simulink model "wall_plumbing_V2"  (R2017b)
settings: Solver=VariableStepAuto  StartTime=0.0  StopTime=tf  RelTol=1e-3  AbsTol=1e-3  EnableMultiTasking=on
values from neighbouring files (symbols this model uses):
  cistern_diam = 100    [plumbing_variables.m]
  cistern_inlet_diam = 2    [plumbing_variables.m]
  cistern_outlet_diam = 2    [plumbing_variables.m]
  random_seed = rand()    [plumbing_variables.m]
  swh_inlet_diam = 2    [plumbing_variables.m]
  swh_outlet_diam = 2    [plumbing_variables.m]
undefined symbols (not defined in the file or in its folder): sigbuilder_block
libraries: fl_lib x59, nesl_utility x42, sh_lib x12, simulink x5, SimscapeFluids_lib x1
(part 1 of 2)
settings Model: Creator=solan  LastModifiedBy=solan
settings SolverCC: ZeroCrossAlgorithm=Adaptive  AlgebraicLoopSolver=LineSearch
settings DataIOCC: LimitDataPoints=on  MaxDataPoints=10000
settings OptimizationCC: LifeSpan=inf
settings DebuggingCC: AllowSymbolicDim=off  SFUnexpectedBacktrackingDiag=warning  SFNoUnconditionalDefaultTransitionDiag=warning  SFExecutionAtInitializationDiag=none
settings CodeAppCC: StateflowObjectComments=on
settings GRTTargetCC: TargetLangStandard=C89/C90 (ANSI)  GeneratePreprocessorConditionals=Disable all
settings ConfigComp: CovMetricSettings=dw  CovHtmlReporting=on  CovSaveCumulativeToWorkspaceVar=on  CovSaveSingleToWorkspaceVar=on  CovExternalEMLEnable=off  CovSFcnEnable=off
settings SimscapeCC: SimscapeLogType=all  SimscapeLogSimulationStatistics=on  SimscapeLogOpenViewer=on  SimscapeLogDataHistory=10000

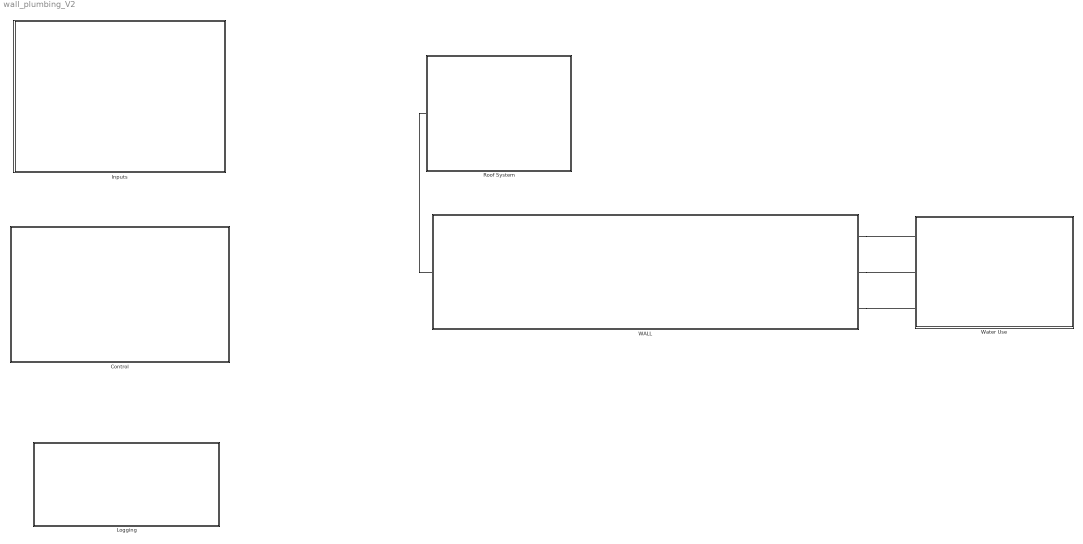
== system wall_plumbing_V2 ==
  Control : Subsystem
  Inputs : Subsystem
  Logging : Subsystem
  Roof System : Subsystem
  WALL : Subsystem
  Water Use : Subsystem
  connections:
  WALL/RConn2 -- Water Use/LConn2
  WALL/RConn1 -- Water Use/LConn1
  Roof System/LConn1 -- WALL/LConn1
  WALL/RConn3 -- Water Use/LConn3

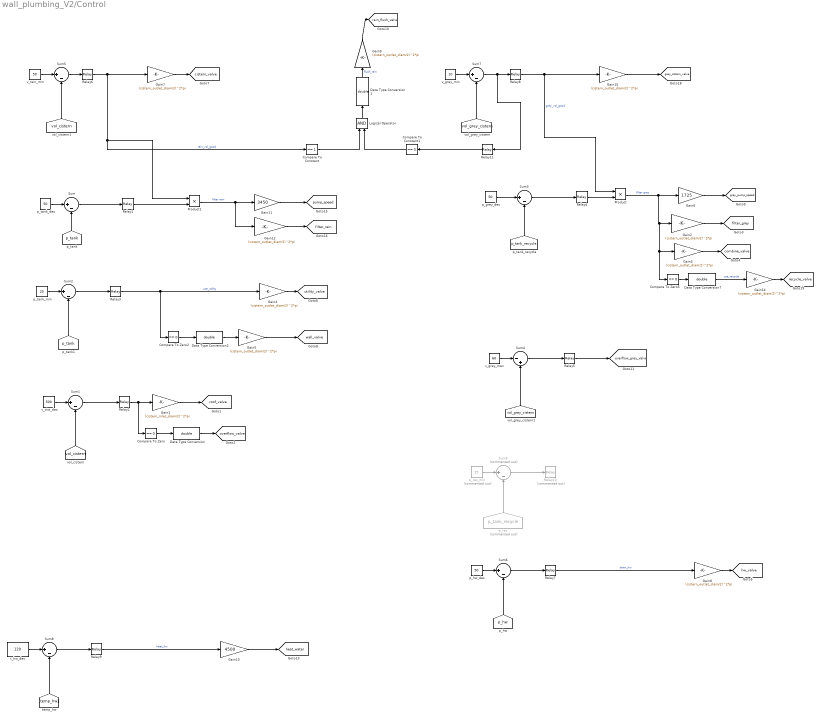
== system wall_plumbing_V2/Control ==
  Compare To Constant : simulink/Logic and Bit Operations/Compare To Constant  relop===  const=1  OutDataTypeStr=boolean
  Compare To Constant1 : simulink/Logic and Bit Operations/Compare To Constant  relop===  const=0  OutDataTypeStr=boolean
  Compare To Zero : simulink/Logic and Bit Operations/Compare To Zero  relop===  OutDataTypeStr=boolean
  Compare To Zero2 : simulink/Logic and Bit Operations/Compare To Zero  relop===  OutDataTypeStr=boolean
  Compare To Zero5 : simulink/Logic and Bit Operations/Compare To Zero  relop===  OutDataTypeStr=boolean
  Data Type Conversion{,1..2,7} (4 alike) : DataTypeConversion  OutDataTypeStr=double
  Gain1 : Gain  Gain=(cistern_inlet_diam/2)^2*pi
  Gain10 : Gain  Gain=4500
  Gain11 : Gain  Gain=3450
  Gain{2..5,7..9,12,14..15} (10 alike) : Gain  Gain=(cistern_outlet_diam/2)^2*pi
  Gain6 : Gain  Gain=1725
  Logical Operator : Logic  AllPortsSameDT=off  OutDataTypeStr=boolean
  Product : Product
  Product1 : Product
  Relay1 : Relay  OnSwitchValue=10  OffSwitchValue=-10
  Relay10 : Relay  Commented=on  OnSwitchValue=4  OffSwitchValue=-5  OnOutputValue=0  OffOutputValue=1
  Relay11 : Relay  OnSwitchValue=-5  OffSwitchValue=-20  OnOutputValue=0  OffOutputValue=1
  Relay2 : Relay  OnSwitchValue=25  OffSwitchValue=-25
  Relay3 : Relay  OnSwitchValue=4  OffSwitchValue=-5
  Relay4 : Relay  OnSwitchValue=5  OffSwitchValue=-5
  Relay5 : Relay  OnSwitchValue=5  OffSwitchValue=-5
  Relay6 : Relay  OnSwitchValue=5  OffSwitchValue=-5  OnOutputValue=0  OffOutputValue=1
  Relay7 : Relay  OnSwitchValue=10  OffSwitchValue=-10
  Relay8 : Relay  OnSwitchValue=5  OffSwitchValue=-5  OnOutputValue=0  OffOutputValue=1
  Relay9 : Relay  OnSwitchValue=10  OffSwitchValue=-10
  Sum{,1..3,5..8} (8 alike) : Sum  Inputs=|+-
  Sum4 : Sum  Inputs=|-+
  Sum9 : Sum  Commented=on  Inputs=|+-
  p_grey_des : Constant  Value=50
  p_hw_des : Constant  Value=50
  p_rec : From  Commented=on  GotoTag=p_tank_recycle  TagVisibility=global
  p_rec_min : Constant  Commented=on  Value=25
  p_tank_des : Constant  Value=50
  p_tank_min : Constant  Value=25
  t_hw_des : Constant  Value=120
  v_cist_des : Constant  Value=500
  v_grey_max : Constant  Value=60
  v_grey_min : Constant  Value=10
  v_rain_min : Constant  Value=50
  tag scope: cistern_valve=global, combine_valve=global, filter_grey=global, filter_rain=global, grey_cistern_valve=global, grey_pump_speed=global, heat_water=global, hw_valve=global, overflow_grey_valve=global, overflow_valve=global, pump_speed=global, rain_flush_valve=global, recycle_valve=global, roof_valve=global, utility_valve=global, wall_valve=global
  wires:
  p_tank_des/1 -> Sum/1
  [p_tank] -> Sum/2
  [vol_cistern] -> Sum1/2
  v_cist_des/1 -> Sum1/1
  Relay2/1 -> Compare To Zero/1, Gain1/1
  Gain1/1 -> [roof_valve]
  Compare To Zero/1 -> Data Type Conversion/1
  Data Type Conversion/1 -> [overflow_valve]
  [p_tank] -> Sum2/2
  Gain4/1 -> [utility_valve]
  p_tank_min/1 -> Sum2/1
  Gain5/1 -> [wall_valve]
  Relay4/1 -> Product/2
  [p_tank_recycle] -> Sum3/2
  p_grey_des/1 -> Sum3/1
  Relay1/1 -> Product1/2
  Gain11/1 -> [pump_speed]
  Product1/1 -> Gain12/1, Gain11/1  "filter rain"
  Gain12/1 -> [filter_rain]
  Relay3/1 -> Compare To Zero2/1, Gain4/1  "use_utility"
  Product/1 -> Compare To Zero5/1, Gain3/1, Gain2/1, Gain6/1  "filter grey"
  Gain6/1 -> [grey_pump_speed]
  Gain2/1 -> [filter_grey]
  Sum2/1 -> Relay3/1
  Sum/1 -> Relay1/1
  Sum1/1 -> Relay2/1
  Sum3/1 -> Relay4/1
  Gain3/1 -> [combine_valve]
  Compare To Zero5/1 -> Data Type Conversion7/1
  Data Type Conversion7/1 -> Gain14/1  "use_recycle"
  Gain14/1 -> [recycle_valve]
  [vol_grey_cistern] -> Sum4/2
  v_grey_max/1 -> Sum4/1
  Sum4/1 -> Relay5/1
  Relay5/1 -> [overflow_grey_valve]
  Compare To Zero2/1 -> Data Type Conversion2/1
  Data Type Conversion2/1 -> Gain5/1
  Relay6/1 -> Compare To Constant/1, Product1/1, Gain7/1  "rain_vol_good"
  v_rain_min/1 -> Sum5/1
  Gain7/1 -> [cistern_valve]
  [vol_cistern] -> Sum5/2
  Sum5/1 -> Relay6/1
  Relay8/1 -> Product/1, Gain15/1  "grey_vol_good"
  v_grey_min/1 -> Sum7/1
  Gain15/1 -> [grey_cistern_valve]
  [vol_grey_cistern] -> Sum7/2
  Sum7/1 -> Relay11/1, Relay8/1
  Gain8/1 -> [hw_valve]
  p_hw_des/1 -> Sum6/1
  [p_hw] -> Sum6/2
  Sum6/1 -> Relay7/1
  Relay9/1 -> Gain10/1  "heat_hw"
  Gain10/1 -> [heat_water]
  [temp_hw] -> Sum8/2
  Sum8/1 -> Relay9/1
  t_hw_des/1 -> Sum8/1
  p_rec_min/1 -> Sum9/1
  p_rec/1 -> Sum9/2
  Sum9/1 -> Relay10/1
  Relay7/1 -> Gain8/1  "draw_hw"
  Compare To Constant/1 -> Logical Operator/1
  Compare To Constant1/1 -> Logical Operator/2
  Gain9/1 -> [rain_flush_valve]
  Logical Operator/1 -> Data Type Conversion1/1
  Data Type Conversion1/1 -> Gain9/1  "flush_rain"
  Relay11/1 -> Compare To Constant1/1

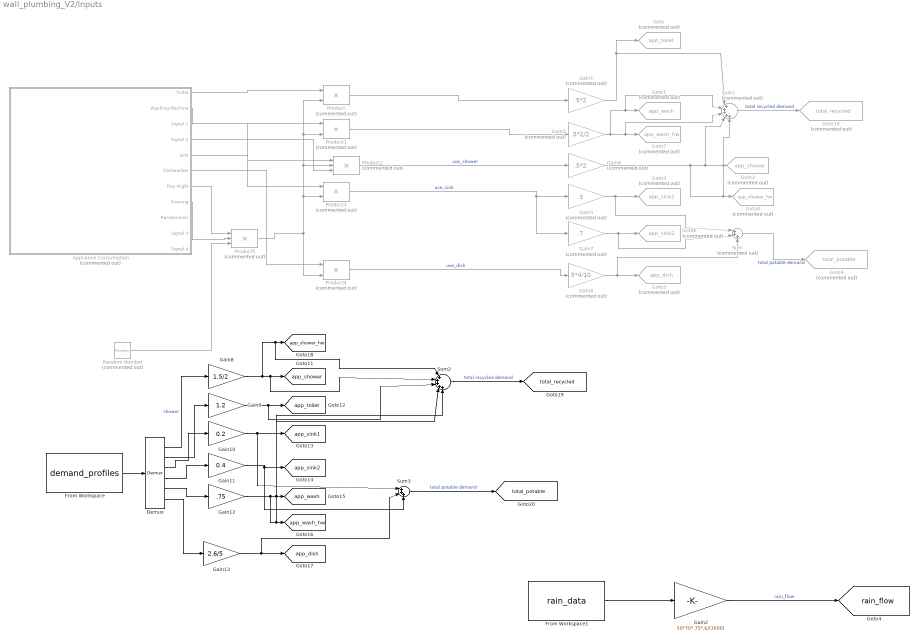
== system wall_plumbing_V2/Inputs ==
  Appliance Consumption : Subsystem  Tag=STV Subsys  Commented=on  LoadFcn=sigbuilder_block('load');  StartFcn=sigbuilder_block('start');  StopFcn=sigbuilder_block('stop');  ClipboardFcn=sigbuilder_block('clipboard');  mask(Sigbuilder block){tuvar=[0:10]}
      mask help: Simulink:masks:SigbuilderBlock_MD
      mask init:
      | if ~strcmp(get_param(bdroot(gcbh),'SimulationStatus'),'stopped') tuvar = sigbuilder_block('maskInit'); end
      settings: CopyFcn=sigbuilder_block('copy');  DeleteFcn=sigbuilder_block('delete');  ModelCloseFcn=sigbuilder_block('modelClose');  PreSaveFcn=sigbuilder_block('preSave');  PauseFcn=sigbuilder_block('pause');  ContinueFcn=sigbuilder_block('continue');  NameChangeFcn=sigbuilder_block('namechange');  OpenFcn=sigbuilder_block('open',[348 246 1517 1004 ]);  CloseFcn=sigbuilder_block('close');
      mask Display: plot(0, 0, 100, 100,[2, 2, 32, 32, 2], [68, 8, 8, 68, 68],[32, 2], [38, 38], [32, 19, 2],[53, 60, 44], [32, 17, 17, 2],[16, 16, 31, 31]);txt = getActiveGroup(gcbh);text(2, 100, txt,'verticalAlignment', 'top');
  Demux : Demux  Outputs=6
  From Workspace : FromWorkspace  VariableName=demand_profiles  SampleTime=0
  From Workspace1 : FromWorkspace  VariableName=rain_data  SampleTime=0  Interpolate=off  OutputAfterFinalValue=Setting to zero
  Gain1 : Gain  Commented=on  Gain=.5*2
  Gain10 : Gain  Gain=0.2
  Gain11 : Gain  Gain=0.4
  Gain12 : Gain  Gain=.75
  Gain13 : Gain  Gain=2.6/5
  Gain2 : Gain  Gain=50*70*.75*.6/(3600)
  Gain3 : Gain  Commented=on  Gain=.5*2/2
  Gain4 : Gain  Commented=on  Gain=.5*2
  Gain5 : Gain  Commented=on  Gain=.3
  Gain6 : Gain  Commented=on  Gain=.5*4/10
  Gain7 : Gain  Commented=on  Gain=.7
  Gain8 : Gain  Gain=1.5/2
  Gain9 : Gain  Gain=1.2
  Goto : Goto  Commented=on  GotoTag=app_toilet  TagVisibility=global
  Goto1 : Goto  Commented=on  GotoTag=app_wash  TagVisibility=global
  Goto10 : Goto  Commented=on  GotoTag=total_recycled  TagVisibility=global
  Goto2 : Goto  Commented=on  GotoTag=app_shower  TagVisibility=global
  Goto3 : Goto  Commented=on  GotoTag=app_sink1  TagVisibility=global
  Goto5 : Goto  Commented=on  GotoTag=app_dish  TagVisibility=global
  Goto6 : Goto  Commented=on  GotoTag=app_sink2  TagVisibility=global
  Goto7 : Goto  Commented=on  GotoTag=app_wash_hw  TagVisibility=global
  Goto8 : Goto  Commented=on  GotoTag=app_shower_hw  TagVisibility=global
  Goto9 : Goto  Commented=on  GotoTag=total_potable  TagVisibility=global
  Product{,1,3..4} (4 alike) : Product  Commented=on
  Product2 : Product  Commented=on  Inputs=3
  Product5 : Product  Commented=on  Inputs=3
  Random Number : RandomNumber  Commented=on  Mean=1  Variance=0.1  Seed=random_seed  SampleTime=5*60
  Sum : Sum  Commented=on  Inputs=|+++
  Sum1 : Sum  Commented=on  Inputs=|+++++
  Sum2 : Sum  Inputs=|+++++
  Sum3 : Sum  Inputs=|+++
  tag scope: app_dish=global, app_shower=global, app_shower_hw=global, app_sink1=global, app_sink2=global, app_toilet=global, app_wash=global, app_wash_hw=global, rain_flow=global, total_potable=global, total_recycled=global
  wires:
  From Workspace1/1 -> Gain2/1
  Gain2/1 -> [rain_flow]  "rain_flow"
  Product5/1 -> Product3/2, Product1/2, Product/2, Product2/2, Product4/2
  Gain1/1 -> Sum1/1, Goto/1
  Gain3/1 -> Sum1/3, Goto7/1, Sum1/2, Goto1/1
  Gain4/1 -> Sum1/5, Goto8/1, Sum1/4, Goto2/1
  Gain5/1 -> Sum/1, Goto3/1
  Gain6/1 -> Sum/3, Goto5/1
  Gain7/1 -> Sum/2, Goto6/1
  Sum/1 -> Goto9/1  "total potable demand"
  Sum1/1 -> Goto10/1  "total recycled demand"
  Appliance Consumption/6(Dishwasher) -> Product4/1
  Appliance Consumption/2(Washing Machine) -> Product1/1
  Appliance Consumption/3(Signal 1) -> Product2/1
  Appliance Consumption/4(Signal 2) -> Product2/3
  Appliance Consumption/1(Toilet) -> Product/1
  Appliance Consumption/7(Day-Night) -> Product5/1
  Product3/1 -> Gain7/1, Gain5/1  "use_sink"
  Product2/1 -> Gain4/1  "use_shower"
  Product1/1 -> Gain3/1
  Product/1 -> Gain1/1
  Product4/1 -> Gain6/1  "use_dish"
  Appliance Consumption/8(Evening) -> Product5/2
  Appliance Consumption/5(Sink) -> Product3/1
  Random Number/1 -> Product5/3
  From Workspace/1 -> Demux/1
  Demux/1 -> Gain8/1  "shower"
  Gain8/1 -> Sum2/1, [app_shower_hw], Sum2/2, [app_shower]
  Demux/2 -> Gain9/1
  Gain9/1 -> Sum2/3, [app_toilet]
  Demux/3 -> Gain10/1
  Gain10/1 -> Sum3/1, [app_sink1]
  Demux/4 -> Gain11/1
  Gain11/1 -> Sum3/3, [app_sink2]
  Gain12/1 -> Sum2/5, [app_wash_hw], Sum2/4, [app_wash]
  Demux/5 -> Gain12/1
  Demux/6 -> Gain13/1
  Gain13/1 -> Sum3/2, [app_dish]
  Sum2/1 -> [total_recycled]  "total recycled demand"
  Sum3/1 -> [total_potable]  "total potable demand"

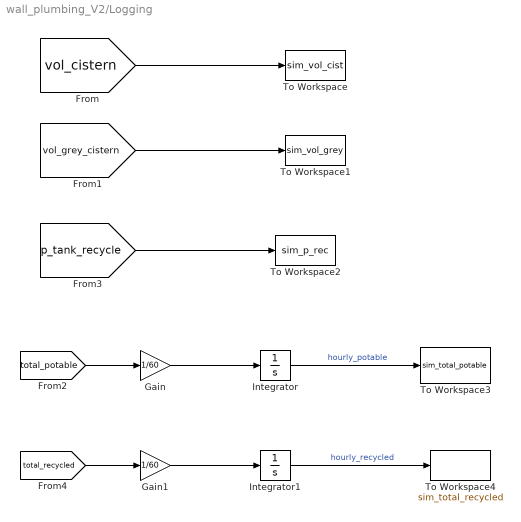
== system wall_plumbing_V2/Logging ==
  Gain : Gain  Gain=1/60
  Gain1 : Gain  Gain=1/60
  Integrator : Integrator
  Integrator1 : Integrator
  To Workspace : ToWorkspace  VariableName=sim_vol_cist  SaveFormat=Timeseries  SampleTime=3600
  To Workspace1 : ToWorkspace  VariableName=sim_vol_grey  SaveFormat=Timeseries  SampleTime=3600
  To Workspace2 : ToWorkspace  VariableName=sim_p_rec  SaveFormat=Timeseries  SampleTime=3600
  To Workspace3 : ToWorkspace  VariableName=sim_total_potable  SaveFormat=Timeseries  SampleTime=3600
  To Workspace4 : ToWorkspace  VariableName=sim_total_recycled  SaveFormat=Timeseries  SampleTime=3600
  wires:
  [vol_cistern] -> To Workspace/1
  [vol_grey_cistern] -> To Workspace1/1
  [p_tank_recycle] -> To Workspace2/1
  [total_potable] -> Gain/1
  [total_recycled] -> Gain1/1
  Integrator1/1 -> To Workspace4/1  "hourly_recycled"
  Integrator/1 -> To Workspace3/1  "hourly_potable"
  Gain/1 -> Integrator/1
  Gain1/1 -> Integrator1/1

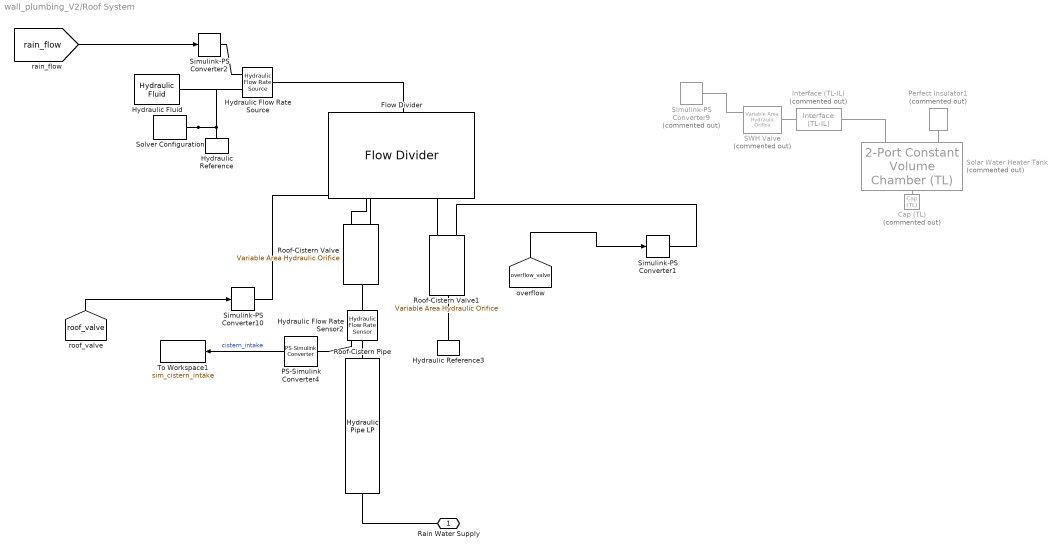
== system wall_plumbing_V2/Roof System ==
  Cap (TL) : fl_lib/Thermal Liquid/Elements/Cap (TL)  Commented=on  p_specify=off  p_priority=None  p=0.101325 MPa  p_nominal_specify=off  p_nominal_unit=MPa  p_nominal_value=1  T_specify=off  T_priority=None  T=293.15 K  T_nominal_specify=off  T_nominal_unit=K  T_nominal_value=1
      settings: SourceProductName=Simscape  SourceProductBaseCode=SS
  Flow Divider : sh_lib/Valves/Flow Control Valves/Flow Divider  area_A=1e-4 m^2  area_B=1e-4 m^2  C_d_A=0.7  C_d_B=0.7  lam_spec=1  B_lam_A=0.999  B_lam_B=0.999  Re_cr_A=10  Re_cr_B=10  orifice_d=0.005 m  orifice_numb=4  C_d_or=0.65  init_A=0.0025 m  init_B=0.0025 m  leak_area=1e-9 m^2  lam_spec_or=1  B_lam_or_A=0.999  B_lam_or_B=0.999  Re_cr_or_A=10  Re_cr_or_B=10  area_sc=1.6e-4 m^2  stroke=0.005 m  spring_rate=1e3 N/m  damping=150 N/(m/s)  stop_coefficient=1e12 s*N/m^2
      settings: SourceProductName=Simscape Fluids  SourceProductBaseCode=SH
  Hydraulic Flow Rate Sensor2 : fl_lib/Hydraulic/Hydraulic Sensors/Hydraulic Flow Rate Sensor
      settings: SourceProductName=Simscape
  Hydraulic Flow Rate Source : fl_lib/Hydraulic/Hydraulic Sources/Hydraulic Flow Rate Source
      settings: SourceProductName=Simscape  SourceProductBaseCode=SS
  Hydraulic Fluid : sh_lib/Hydraulic Utilities/Hydraulic Fluid  DataSource=1  SelFluid=24  SysTemp=15  TrapAir=0.005  ViscDerFactor=1  range_error=2
      settings: SourceProductName=Simscape Fluids
  Hydraulic Reference : fl_lib/Hydraulic/Hydraulic Elements/Hydraulic Reference
      settings: SourceProductName=Foundation Library
  Hydraulic Reference3 : fl_lib/Hydraulic/Hydraulic Elements/Hydraulic Reference
      settings: SourceProductName=Foundation Library
  Interface (TL-IL) : SimscapeFluids_lib/Fluid Network Interfaces/Interface (TL-IL)  Commented=on  T_B=293.15 K  area=0.01 m^2
      settings: SourceProductName=Simscape Fluids  SourceProductBaseCode=SH
  PS-Simulink Converter4 : nesl_utility/PS-Simulink Converter  PhysicalDomain=network_engine_domain  SubClassName=ps_output  LeftPortType=input  RightPortType=output  PseudoPeriodic=off  Frequencies=[]  Unit=gal/min  AffineConversion=off
  Perfect Insulator1 : fl_lib/Thermal/Thermal Elements/Perfect Insulator  Commented=on  T_specify=off  T_priority=None  T=0 K  T_nominal_specify=off  T_nominal_unit=K  T_nominal_value=1
      settings: SourceProductName=Simscape
  Roof-Cistern Pipe : sh_lib/Low-Pressure Blocks/Hydraulic Pipe LP  cs_type=1  d_in=cistern_inlet_diam in  area=1e-4 m^2  D_h=1.12e-2 m  s_factor=64  length=roof_cistern_pipe_length ft  length_ad=1 m  roughness=15e-6 m  Re_lam=2000  Re_turb=4000  elevation_A=roof_height ft  elevation_B=cistern_inlet_height ft  g=9.80665 m/s^2  wall_type=1  pr_r_coef=2e-12 m/Pa  time_const=0.01 s  k_sh=1.4  p0=0 Pa
      settings: SourceProductName=Simscape Fluids  SourceProductBaseCode=SH
  Roof-Cistern Valve : fl_lib/Hydraulic/Hydraulic Elements/Variable Area Hydraulic Orifice  C_d=0.7  min_area=1e-12 m^2  lam_spec=1  B_lam=0.999  Re_cr=12  q_specify=off  q_priority=None  q=0.001 m^3/s  q_nominal_specify=off  q_nominal_unit=m^3/s  q_nominal_value=1  p_specify=off  p_priority=None  p=0 Pa  p_nominal_specify=off  p_nominal_unit=Pa  p_nominal_value=1
      settings: SourceProductName=Simscape  SourceProductBaseCode=SS
  Roof-Cistern Valve1 : fl_lib/Hydraulic/Hydraulic Elements/Variable Area Hydraulic Orifice  C_d=0.7  min_area=1e-12 m^2  lam_spec=1  B_lam=0.999  Re_cr=12  q_specify=off  q_priority=None  q=0.001 m^3/s  q_nominal_specify=off  q_nominal_unit=m^3/s  q_nominal_value=1  p_specify=off  p_priority=None  p=0 Pa  p_nominal_specify=off  p_nominal_unit=Pa  p_nominal_value=1
      settings: SourceProductName=Simscape  SourceProductBaseCode=SS
  SWH Valve : fl_lib/Hydraulic/Hydraulic Elements/Variable Area Hydraulic Orifice  Commented=on  C_d=0.7  min_area=1e-12 m^2  lam_spec=1  B_lam=0.999  Re_cr=12  q_specify=off  q_priority=None  q=0.001 m^3/s  q_nominal_specify=off  q_nominal_unit=m^3/s  q_nominal_value=1  p_specify=off  p_priority=None  p=0 Pa  p_nominal_specify=off  p_nominal_unit=Pa  p_nominal_value=1
      settings: SourceProductName=Simscape  SourceProductBaseCode=SS
  Simulink-PS Converter1 : nesl_utility/Simulink-PS Converter  PhysicalDomain=network_engine_domain  SubClassName=ps_input  LeftPortType=input  RightPortType=output  PseudoPeriodic=off  Frequencies=[]  NoiseDistribution=none  NoiseParameters=[]  Unit=1  AffineConversion=off  FilteringAndDerivatives=zero  SimscapeFilterOrder=1  InputFilterTimeConstant=0.001  UdotUserProvided=1
  Simulink-PS Converter10 : nesl_utility/Simulink-PS Converter  PhysicalDomain=network_engine_domain  SubClassName=ps_input  LeftPortType=input  RightPortType=output  PseudoPeriodic=off  Frequencies=[]  NoiseDistribution=none  NoiseParameters=[]  Unit=in^2  AffineConversion=off  FilteringAndDerivatives=zero  SimscapeFilterOrder=1  InputFilterTimeConstant=0.001  UdotUserProvided=1
  Simulink-PS Converter2 : nesl_utility/Simulink-PS Converter  PhysicalDomain=network_engine_domain  SubClassName=ps_input  LeftPortType=input  RightPortType=output  PseudoPeriodic=off  Frequencies=[]  NoiseDistribution=none  NoiseParameters=[]  Unit=gal/s  AffineConversion=off  FilteringAndDerivatives=zero  SimscapeFilterOrder=1  InputFilterTimeConstant=0.001  UdotUserProvided=1
  Simulink-PS Converter9 : nesl_utility/Simulink-PS Converter  Commented=on  PhysicalDomain=network_engine_domain  SubClassName=ps_input  LeftPortType=input  RightPortType=output  PseudoPeriodic=off  Frequencies=[]  NoiseDistribution=none  NoiseParameters=[]  Unit=1  AffineConversion=off  FilteringAndDerivatives=zero  SimscapeFilterOrder=1  InputFilterTimeConstant=0.001  UdotUserProvided=1
  Solar Water Heater Tank : fl_lib/Thermal Liquid/Elements/2-Port Constant Volume Chamber (TL)  Commented=on  volume=swh_volume gal  area_A=3.14*(swh_inlet_diam/2)^2 in^2  area_B=3.14*(swh_outlet_diam/2)^2 in^2  p_chamber_specify=off  p_chamber_priority=High  p_chamber=0.101325 MPa  p_chamber_nominal_specify=off  p_chamber_nominal_unit=MPa  p_chamber_nominal_value=1  T_chamber_specify=off  T_chamber_priority=High  T_chamber=293.15 K  T_chamber_nominal_specify=off  T_chamber_nominal_unit=K  T_chamber_nominal_value=1  u_chamber_specify=off  u_chamber_priority=None  u_chamber=83.90600000000001 kJ/kg  u_chamber_nominal_specify=off  u_chamber_nominal_unit=kJ/kg  u_chamber_nominal_value=1  rho_specify=off  rho_priority=None  rho=998.21 kg/m^3  rho_nominal_specify=off  rho_nominal_unit=kg/m^3  rho_nominal_value=1
      settings: SourceProductName=Simscape  SourceProductBaseCode=SS
  Solver Configuration : nesl_utility/Solver Configuration  PhysicalDomain=network_engine_domain  SubClassName=solver  LeftPortType=input  RightPortType=generic  Accelerate=off  Tones=[]  Harmonics=[]  SimulateNoise=off  Profile=off  UseLocalSampling=off  EnableSwitchedLinearOptims=on  FrequencyDomain=off  UseCCode=off  RelTol=0.001  AbsTol=1e-06  MinStep=1e-09  ToWorkspace=off  RevertToSquareIcSolve=off  NumHomotopyIterations=100  PhasorMode=off  PhasorModeNumHarmonics=1  DoDC=off  ResidualTolerance=1e-09  UseLocalSolver=off  LocalSolverChoice=NE_BACKWARD_EULER_ADVANCER  LocalSolverSampleTime=0.001  DoFixedCost=off  MaxNonlinIter=3  MaxModeIter=2  LinearAlgebra=Sparse  DelaysMemoryBudget=1024  AutomaticFiltering=on  FilteringTimeConstant=0.001
  To Workspace1 : ToWorkspace  VariableName=sim_cistern_intake  SaveFormat=Timeseries  SampleTime=-1
  Rain Water Supply : PMIOPort  Port=1  Side=Left
  wires:
  [rain_flow] -> Simulink-PS Converter2/1
  [roof_valve] -> Simulink-PS Converter10/1
  [overflow_valve] -> Simulink-PS Converter1/1
  PS-Simulink Converter4/1 -> To Workspace1/1  "cistern_intake"
  connections:
  Solver Configuration/RConn1 -- Hydraulic Flow Rate Source/RConn2 -- Hydraulic Fluid/RConn1 -- Hydraulic Reference/LConn1
  SWH Valve/RConn1 -- Interface (TL-IL)/RConn1
  Interface (TL-IL)/LConn1 -- Solar Water Heater Tank/LConn1
  Hydraulic Flow Rate Source/RConn1 -- Simulink-PS Converter2/RConn1
  Cap (TL)/LConn1 -- Solar Water Heater Tank/RConn1
  Perfect Insulator1/LConn1 -- Solar Water Heater Tank/LConn2
  Simulink-PS Converter9/RConn1 -- SWH Valve/LConn1
  Simulink-PS Converter10/RConn1 -- Roof-Cistern Valve/LConn1
  Flow Divider/RConn2 -- Roof-Cistern Valve/LConn2
  Hydraulic Reference3/LConn1 -- Roof-Cistern Valve1/RConn1
  Roof-Cistern Valve1/LConn2 -- Flow Divider/RConn1
  Simulink-PS Converter1/RConn1 -- Roof-Cistern Valve1/LConn1
  Flow Divider/LConn1 -- Hydraulic Flow Rate Source/LConn1
  PS-Simulink Converter4/LConn1 -- Hydraulic Flow Rate Sensor2/RConn1
  Hydraulic Flow Rate Sensor2/LConn1 -- Roof-Cistern Valve/RConn1
  Roof-Cistern Pipe/LConn1 -- Hydraulic Flow Rate Sensor2/RConn2
  Roof-Cistern Pipe/RConn1 -- Rain Water Supply/RConn1

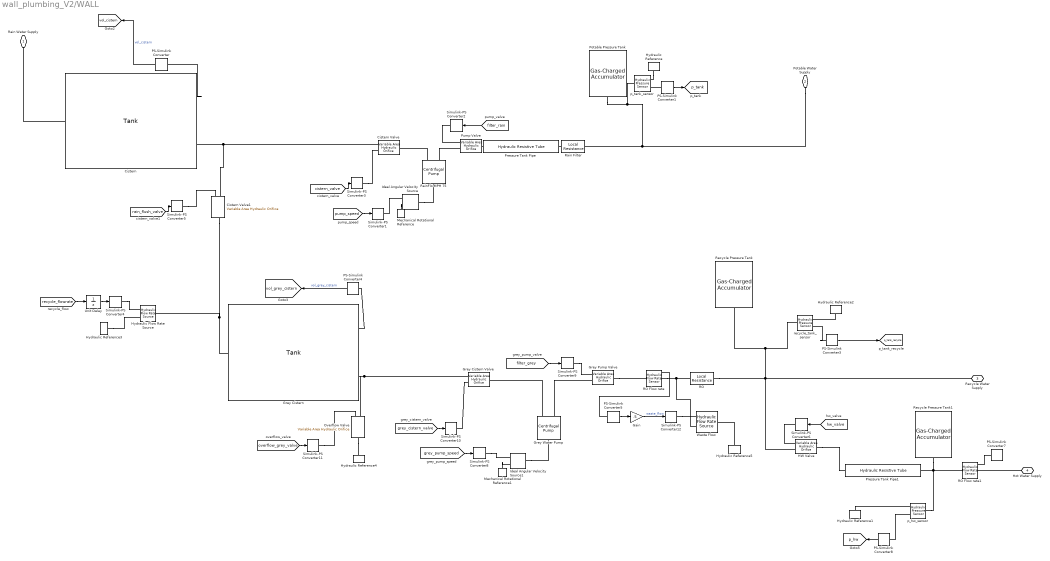
== system wall_plumbing_V2/WALL ==
  Cistern : sh_lib/Low-Pressure Blocks/Tank  press=0 Pa  level_spec=1  tank_area=3.14*(cistern_diam/2)^2 in^2  fluid_volume_tab=[0, .0028, .0065, .0114, .0176, .0252, .0344, .0436, .0512, .0574, .0623, .066, .0688, .0707, .072, .0727] m^3  fluid_level_tab=[0, .02, .04, .06, .08, .1, .12, .14, .16, .18, .2, .22, .24, .26, .28, .3] m  interp_method=1  extrap_method=1  pipe_diam=0.02 m  loss_coeff=1.2  g=9.80665 m/s^2  min_level=1e-3 m  fluid_level_check=0  volume_specify=on  volume_priority=High  volume=480 gal  volume_nominal_specify=off  volume_nominal_unit=l  volume_nominal_value=1  level_specify=off  level_priority=None  level=0.025 m  level_nominal_specify=off  level_nominal_unit=m  level_nominal_value=1  pipe_diam_A=cistern_outlet_diam in  loss_coeff_A=1.2  height_B=cistern_inlet_height ft  pipe_diam_B=cistern_inlet_diam in  loss_coeff_B=1.2  height_C=0.8 m  pipe_diam_C=0.02 m  loss_coeff_C=1.2
      settings: SourceProductName=Simscape Fluids  SourceProductBaseCode=SH
  Cistern Valve : fl_lib/Hydraulic/Hydraulic Elements/Variable Area Hydraulic Orifice  C_d=0.7  min_area=1e-12 m^2  lam_spec=1  B_lam=0.999  Re_cr=12  q_specify=off  q_priority=None  q=0.001 m^3/s  q_nominal_specify=off  q_nominal_unit=m^3/s  q_nominal_value=1  p_specify=off  p_priority=None  p=0 Pa  p_nominal_specify=off  p_nominal_unit=Pa  p_nominal_value=1
      settings: SourceProductName=Simscape  SourceProductBaseCode=SS
  Cistern Valve1 : fl_lib/Hydraulic/Hydraulic Elements/Variable Area Hydraulic Orifice  C_d=0.7  min_area=1e-12 m^2  lam_spec=1  B_lam=0.999  Re_cr=12  q_specify=off  q_priority=None  q=0.001 m^3/s  q_nominal_specify=off  q_nominal_unit=m^3/s  q_nominal_value=1  p_specify=off  p_priority=None  p=0 Pa  p_nominal_specify=off  p_nominal_unit=Pa  p_nominal_value=1
      settings: SourceProductName=Simscape  SourceProductBaseCode=SS
  Gain : Gain  Gain=.5
  Grey Cistern : sh_lib/Low-Pressure Blocks/Tank  press=0 Pa  level_spec=1  tank_area=3.14*(.25)^2 m^2  fluid_volume_tab=[0, .0028, .0065, .0114, .0176, .0252, .0344, .0436, .0512, .0574, .0623, .066, .0688, .0707, .072, .0727] m^3  fluid_level_tab=[0, .02, .04, .06, .08, .1, .12, .14, .16, .18, .2, .22, .24, .26, .28, .3] m  interp_method=1  extrap_method=1  pipe_diam=0.02 m  loss_coeff=1.2  g=9.80665 m/s^2  min_level=1e-3 m  fluid_level_check=0  volume_specify=on  volume_priority=High  volume=50 gal  volume_nominal_specify=off  volume_nominal_unit=l  volume_nominal_value=1  level_specify=off  level_priority=None  level=0.025 m  level_nominal_specify=off  level_nominal_unit=m  level_nominal_value=1  pipe_diam_A=cistern_outlet_diam in  loss_coeff_A=1.2  height_B=1 m  pipe_diam_B=cistern_inlet_diam in  loss_coeff_B=1.2  height_C=0.8 m  pipe_diam_C=0.02 m  loss_coeff_C=1.2
      settings: SourceProductName=Simscape Fluids  SourceProductBaseCode=SH
  Grey Cistern Valve : fl_lib/Hydraulic/Hydraulic Elements/Variable Area Hydraulic Orifice  C_d=0.7  min_area=1e-12 m^2  lam_spec=1  B_lam=0.999  Re_cr=12  q_specify=off  q_priority=None  q=0.001 m^3/s  q_nominal_specify=off  q_nominal_unit=m^3/s  q_nominal_value=1  p_specify=off  p_priority=None  p=0 Pa  p_nominal_specify=off  p_nominal_unit=Pa  p_nominal_value=1
      settings: SourceProductName=Simscape  SourceProductBaseCode=SS
  Grey Pump Valve : fl_lib/Hydraulic/Hydraulic Elements/Variable Area Hydraulic Orifice  C_d=0.7  min_area=1e-12 m^2  lam_spec=1  B_lam=0.999  Re_cr=12  q_specify=off  q_priority=None  q=0.001 m^3/s  q_nominal_specify=off  q_nominal_unit=m^3/s  q_nominal_value=1  p_specify=off  p_priority=None  p=0 Pa  p_nominal_specify=off  p_nominal_unit=Pa  p_nominal_value=1
      settings: SourceProductName=Simscape  SourceProductBaseCode=SS
  Grey Water Pump : sh_lib/Pumps and Motors/Centrifugal Pump  mdl_type=2  c_1=326.8 Pa/(kg/m^3)  c_2=3.104e+4 Pa*s/kg  c_3=1.097e+7 Pa*s^2/(kg*m^3)  c_4=2.136e+5 Pa*s^2/(kg*m^3)  c_f=0.8  design_del=130 lpm  ref_velocity=1.725e+3 rpm  ref_density=940 kg/m^3  leak_resistance=1e+8 Pa/(m^3/s)  T_const=0.1 N*m  trq_press_coeff=1e-6 N*m/Pa  pump_del_1D=1.5*[(29+19)/2 (56+46)/2 (78+68)/2 (109+100)/2 (143+128)/2] gal/hr  press_diff_1D=[250 200 150 100 50] psi  pump_del_power_1D=1.5*[(29+19)/2 (56+46)/2 (78+68)/2 (109+100)/2 (143+128)/2] gal/hr  power_1D=[.28 .28 .245 .225 .165] HP  pump_del_2D=[ 140 125 110 100 80 70 60 50 35 25 15 ] gal/hr  pump_vel_2D=[ 1.69e+3 1.7e+3 1.71e+3 1.725e+3 ] rpm  press_diff_2D=[ 8.300000000000001 8.800000000000001 9.300000000000001 9.9; 7.8 8.300000000000001 8.800000000000001 9.4; 7.2 7.6 8.199999999999999 8.699999999999999; 6.5 7 7.5 8; 5.6 6.1 6.6 7.1; 4.7 5.2 5.7 6.2; 3.4 4 4.4 4.9; 2.3 2.7 3.4 3.6 ] bar  pump_del_power_2D=[ 0 50 100 150 200 250 300 350 ] lpm  power_2D=[ 1.223e+3 1.341e+3 1.467e+3 1.6e+3; 1.414e+3 1.551e+3 1.696e+3 1.85e+3; 1.636e+3 1.794e+3 1.962e+3 2.14e+3; 1.941e+3 2.129e+3 2.326e+3 2.54e+3; 2.224e+3 2.439e+3 2.66e+3 2.91e+3; 2.453e+3 2.691e+3 2.947e+3 3.21e+3; 2.757e+3 3.024e+3 3.307e+3 3.608e+3; 2.945e+3 3.23e+3 3.533e+3 3.854e+3 ] W  interp_method=1  extrap_method=1
      settings: SourceProductName=Simscape Fluids  SourceProductBaseCode=SH
  HW Valve : fl_lib/Hydraulic/Hydraulic Elements/Variable Area Hydraulic Orifice  C_d=0.7  min_area=1e-12 m^2  lam_spec=1  B_lam=0.999  Re_cr=12  q_specify=off  q_priority=None  q=0.001 m^3/s  q_nominal_specify=off  q_nominal_unit=m^3/s  q_nominal_value=1  p_specify=off  p_priority=None  p=0 Pa  p_nominal_specify=off  p_nominal_unit=Pa  p_nominal_value=1
      settings: SourceProductName=Simscape  SourceProductBaseCode=SS
  Hydraulic Flow Rate Source : fl_lib/Hydraulic/Hydraulic Sources/Hydraulic Flow Rate Source
      settings: SourceProductName=Simscape  SourceProductBaseCode=SS
  Hydraulic Reference{,1..5} (6 alike) : fl_lib/Hydraulic/Hydraulic Elements/Hydraulic Reference
      settings: SourceProductName=Foundation Library
  Ideal Angular Velocity Source : fl_lib/Mechanical/Mechanical Sources/Ideal Angular Velocity Source
  Ideal Angular Velocity Source1 : fl_lib/Mechanical/Mechanical Sources/Ideal Angular Velocity Source
  Mechanical Rotational Reference : fl_lib/Mechanical/Rotational Elements/Mechanical Rotational Reference
  Mechanical Rotational Reference1 : fl_lib/Mechanical/Rotational Elements/Mechanical Rotational Reference
  Overflow Valve : fl_lib/Hydraulic/Hydraulic Elements/Variable Area Hydraulic Orifice  C_d=0.7  min_area=1e-12 m^2  lam_spec=1  B_lam=0.999  Re_cr=12  q_specify=off  q_priority=None  q=0.001 m^3/s  q_nominal_specify=off  q_nominal_unit=m^3/s  q_nominal_value=1  p_specify=off  p_priority=None  p=0 Pa  p_nominal_specify=off  p_nominal_unit=Pa  p_nominal_value=1
      settings: SourceProductName=Simscape  SourceProductBaseCode=SS
  PS-Simulink Converter : nesl_utility/PS-Simulink Converter  PhysicalDomain=network_engine_domain  SubClassName=ps_output  LeftPortType=input  RightPortType=output  PseudoPeriodic=off  Frequencies=[]  Unit=gal  AffineConversion=off
  PS-Simulink Converter1 : nesl_utility/PS-Simulink Converter  PhysicalDomain=network_engine_domain  SubClassName=ps_output  LeftPortType=input  RightPortType=output  PseudoPeriodic=off  Frequencies=[]  Unit=psi  AffineConversion=off
  PS-Simulink Converter3 : nesl_utility/PS-Simulink Converter  PhysicalDomain=network_engine_domain  SubClassName=ps_output  LeftPortType=input  RightPortType=output  PseudoPeriodic=off  Frequencies=[]  Unit=psi  AffineConversion=off
  PS-Simulink Converter4 : nesl_utility/PS-Simulink Converter  PhysicalDomain=network_engine_domain  SubClassName=ps_output  LeftPortType=input  RightPortType=output  PseudoPeriodic=off  Frequencies=[]  Unit=gal  AffineConversion=off
  PS-Simulink Converter5 : nesl_utility/PS-Simulink Converter  PhysicalDomain=network_engine_domain  SubClassName=ps_output  LeftPortType=input  RightPortType=output  PseudoPeriodic=off  Frequencies=[]  Unit=gal/min  AffineConversion=off
  PS-Simulink Converter7 : nesl_utility/PS-Simulink Converter  PhysicalDomain=network_engine_domain  SubClassName=ps_output  LeftPortType=input  RightPortType=output  PseudoPeriodic=off  Frequencies=[]  Unit=gal/min  AffineConversion=off
  PS-Simulink Converter8 : nesl_utility/PS-Simulink Converter  PhysicalDomain=network_engine_domain  SubClassName=ps_output  LeftPortType=input  RightPortType=output  PseudoPeriodic=off  Frequencies=[]  Unit=psi  AffineConversion=off
  Potable Pressure Tank : sh_lib/Accumulators/Gas-Charged Accumulator  capacity=5 gal  dead_volume=5*23/140 gal  pr_preload=10 psi  k_sh=1.4  stiff_coeff=1e10 Pa/m^3  penetr_coeff=1e10 s*Pa/m^6  flow_rate_specify=off  flow_rate_priority=None  flow_rate=0.005 m^3/s  flow_rate_nominal_specify=off  flow_rate_nominal_unit=m^3/s  flow_rate_nominal_value=1  liquid_volume_specify=on  liquid_volume_priority=High  liquid_volume=2 gal  liquid_volume_nominal_specify=off  liquid_volume_nominal_unit=m^3  liquid_volume_nominal_value=1  liquid_pressure_specify=off  liquid_pressure_priority=None  liquid_pressure=1.01325e+5 Pa  liquid_pressure_nominal_specify=off  liquid_pressure_nominal_unit=Pa  liquid_pressure_nominal_value=1
      settings: SourceProductName=Simscape Fluids  SourceProductBaseCode=SH
  Pressure Tank Pipe : fl_lib/Hydraulic/Hydraulic Elements/Hydraulic Resistive Tube  cs_type=1  d_in=1/4 in  area=1e-4 m^2  D_h=1.12e-2 m  s_factor=64  length=ptank_pipe_length ft  length_ad=1 m  roughness=15e-6 m  Re_lam=2000  Re_turb=4000  q_specify=off  q_priority=None  q=0.001 m^3/s  q_nominal_specify=off  q_nominal_unit=m^3/s  q_nominal_value=1  p_specify=off  p_priority=None  p=0 Pa  p_nominal_specify=off  p_nominal_unit=Pa  p_nominal_value=1
      settings: SourceProductName=Simscape  SourceProductBaseCode=SS
  Pressure Tank Pipe1 : fl_lib/Hydraulic/Hydraulic Elements/Hydraulic Resistive Tube  cs_type=1  d_in=1/4 in  area=1e-4 m^2  D_h=1.12e-2 m  s_factor=64  length=ptank_pipe_length ft  length_ad=1 m  roughness=15e-6 m  Re_lam=2000  Re_turb=4000  q_specify=off  q_priority=None  q=0.001 m^3/s  q_nominal_specify=off  q_nominal_unit=m^3/s  q_nominal_value=1  p_specify=off  p_priority=None  p=0 Pa  p_nominal_specify=off  p_nominal_unit=Pa  p_nominal_value=1
      settings: SourceProductName=Simscape  SourceProductBaseCode=SS
  Pump Valve : fl_lib/Hydraulic/Hydraulic Elements/Variable Area Hydraulic Orifice  C_d=0.7  min_area=1e-12 m^2  lam_spec=1  B_lam=0.999  Re_cr=12  q_specify=off  q_priority=None  q=0.001 m^3/s  q_nominal_specify=off  q_nominal_unit=m^3/s  q_nominal_value=1  p_specify=off  p_priority=None  p=0 Pa  p_nominal_specify=off  p_nominal_unit=Pa  p_nominal_value=1
      settings: SourceProductName=Simscape  SourceProductBaseCode=SS
  RO : sh_lib/Local Hydraulic Resistances/Local Resistance  area=pi*.125^2 in^2  mdl_type=1  kp_d=2  kp_r=2  lam_spec=1  B_lam=0.999  Re_cr=150  Re_vec=[-4000, -3000, -2000, -1000, -500, -200, -100, -50, -40, -30, -20, -15, -10, 10, 20, 30, 40, 50, 100, 200, 500, 1000, 2000, 4000, 5000, 10000]  loss_coeff_vec=[.25, .3, .65, .9, .65, .75, .9, 1.15, 1.35, 1.65, 2.3, 2.8, 3.1, 5, 2.7, 1.8, 1.46, 1.3, .9, .65, .42, .3, .2, .4, .42, .25]  interp_method=2  extrap_method=2  flow_rate_specify=off  flow_rate_priority=None  flow_rate=0 m^3/s  flow_rate_nominal_specify=off  flow_rate_nominal_unit=m^3/s  flow_rate_nominal_value=1  pressure_drop_specify=off  pressure_drop_priority=None  pressure_drop=0 Pa  pressure_drop_nominal_specify=off  pressure_drop_nominal_unit=Pa  pressure_drop_nominal_value=1
      settings: SourceProductName=Simscape Fluids  SourceProductBaseCode=SH
  RO Flow rate : fl_lib/Hydraulic/Hydraulic Sensors/Hydraulic Flow Rate Sensor
      settings: SourceProductName=Simscape
  RO Flow rate1 : fl_lib/Hydraulic/Hydraulic Sensors/Hydraulic Flow Rate Sensor
      settings: SourceProductName=Simscape
  Rain Filter : sh_lib/Local Hydraulic Resistances/Local Resistance  area=pi*.125^2 in^2  mdl_type=1  kp_d=1.25  kp_r=1.25  lam_spec=1  B_lam=0.999  Re_cr=150  Re_vec=[-4000, -3000, -2000, -1000, -500, -200, -100, -50, -40, -30, -20, -15, -10, 10, 20, 30, 40, 50, 100, 200, 500, 1000, 2000, 4000, 5000, 10000]  loss_coeff_vec=[.25, .3, .65, .9, .65, .75, .9, 1.15, 1.35, 1.65, 2.3, 2.8, 3.1, 5, 2.7, 1.8, 1.46, 1.3, .9, .65, .42, .3, .2, .4, .42, .25]  interp_method=2  extrap_method=2  flow_rate_specify=off  flow_rate_priority=None  flow_rate=0 m^3/s  flow_rate_nominal_specify=off  flow_rate_nominal_unit=m^3/s  flow_rate_nominal_value=1  pressure_drop_specify=off  pressure_drop_priority=None  pressure_drop=0 Pa  pressure_drop_nominal_specify=off  pressure_drop_nominal_unit=Pa  pressure_drop_nominal_value=1
      settings: SourceProductName=Simscape Fluids  SourceProductBaseCode=SH
  RainFlo MPH 75 : sh_lib/Pumps and Motors/Centrifugal Pump  mdl_type=2  c_1=326.8 Pa/(kg/m^3)  c_2=3.104e+4 Pa*s/kg  c_3=1.097e+7 Pa*s^2/(kg*m^3)  c_4=2.136e+5 Pa*s^2/(kg*m^3)  c_f=0.8  design_del=130 lpm  ref_velocity=500 rpm  ref_density=940 kg/m^3  leak_resistance=1e+8 Pa/(m^3/s)  T_const=0.1 N*m  trq_press_coeff=1e-6 N*m/Pa  pump_del_1D=2*[0 6.5 9.2 11.7 14.0 15.8 17.0 18.8 20.2 21.4 22.7 24.0 25.0 26.2 ] gpm  press_diff_1D=[70 65 60 55 50 45 40 35 30 25 20 15 10 5.5 ] psi  pump_del_power_1D="2*[0 7.7 12.9 16.5  22.1 26.2 ] gpm"  power_1D="(0.75/1.7)*[0 7.8e-01   2.1   2.4   2.16   1.7] HP"  pump_del_2D=[ 0 50 100 150 200 250 300 350 ] lpm  pump_vel_2D=[ 3.2e+3 3.3e+3 3.4e+3 3.5e+3 ] rpm  press_diff_2D=[ 8.300000000000001 8.800000000000001 9.300000000000001 9.9; 7.8 8.300000000000001 8.800000000000001 9.4; 7.2 7.6 8.199999999999999 8.699999999999999; 6.5 7 7.5 8; 5.6 6.1 6.6 7.1; 4.7 5.2 5.7 6.2; 3.4 4 4.4 4.9; 2.3 2.7 3.4 3.6 ] bar  pump_del_power_2D=[ 0 50 100 150 200 250 300 350 ] lpm  power_2D=[ 1.223e+3 1.341e+3 1.467e+3 1.6e+3; 1.414e+3 1.551e+3 1.696e+3 1.85e+3; 1.636e+3 1.794e+3 1.962e+3 2.14e+3; 1.941e+3 2.129e+3 2.326e+3 2.54e+3; 2.224e+3 2.439e+3 2.66e+3 2.91e+3; 2.453e+3 2.691e+3 2.947e+3 3.21e+3; 2.757e+3 3.024e+3 3.307e+3 3.608e+3; 2.945e+3 3.23e+3 3.533e+3 3.854e+3 ] W  interp_method=1  extrap_method=1
      settings: SourceProductName=Simscape Fluids  SourceProductBaseCode=SH
  Recycle Pressure Tank : sh_lib/Accumulators/Gas-Charged Accumulator  capacity=140/1.5 gal  dead_volume=23/1.5 gal  pr_preload=10 psi  k_sh=1.4  stiff_coeff=1e10 Pa/m^3  penetr_coeff=1e10 s*Pa/m^6  flow_rate_specify=off  flow_rate_priority=None  flow_rate=0.005 m^3/s  flow_rate_nominal_specify=off  flow_rate_nominal_unit=m^3/s  flow_rate_nominal_value=1  liquid_volume_specify=on  liquid_volume_priority=High  liquid_volume=80/1.5 gal  liquid_volume_nominal_specify=off  liquid_volume_nominal_unit=m^3  liquid_volume_nominal_value=1  liquid_pressure_specify=off  liquid_pressure_priority=None  liquid_pressure=1.01325e+5 Pa  liquid_pressure_nominal_specify=off  liquid_pressure_nominal_unit=Pa  liquid_pressure_nominal_value=1
      settings: SourceProductName=Simscape Fluids  SourceProductBaseCode=SH
  Recycle Pressure Tank1 : sh_lib/Accumulators/Gas-Charged Accumulator  capacity=140/2 gal  dead_volume=23/2 gal  pr_preload=10 psi  k_sh=1.4  stiff_coeff=1e10 Pa/m^3  penetr_coeff=1e10 s*Pa/m^6  flow_rate_specify=off  flow_rate_priority=None  flow_rate=0.005 m^3/s  flow_rate_nominal_specify=off  flow_rate_nominal_unit=m^3/s  flow_rate_nominal_value=1  liquid_volume_specify=on  liquid_volume_priority=High  liquid_volume=40 gal  liquid_volume_nominal_specify=off  liquid_volume_nominal_unit=m^3  liquid_volume_nominal_value=1  liquid_pressure_specify=off  liquid_pressure_priority=None  liquid_pressure=1.01325e+5 Pa  liquid_pressure_nominal_specify=off  liquid_pressure_nominal_unit=Pa  liquid_pressure_nominal_value=1
      settings: SourceProductName=Simscape Fluids  SourceProductBaseCode=SH
  Simulink-PS Converter1 : nesl_utility/Simulink-PS Converter  PhysicalDomain=network_engine_domain  SubClassName=ps_input  LeftPortType=input  RightPortType=output  PseudoPeriodic=off  Frequencies=[]  NoiseDistribution=none  NoiseParameters=[]  Unit=rpm  AffineConversion=off  FilteringAndDerivatives=zero  SimscapeFilterOrder=1  InputFilterTimeConstant=0.001  UdotUserProvided=1
  Simulink-PS Converter{2..3,5..6,9..11} (7 alike) : nesl_utility/Simulink-PS Converter  PhysicalDomain=network_engine_domain  SubClassName=ps_input  LeftPortType=input  RightPortType=output  PseudoPeriodic=off  Frequencies=[]  NoiseDistribution=none  NoiseParameters=[]  Unit=in^2  AffineConversion=off  FilteringAndDerivatives=zero  SimscapeFilterOrder=1  InputFilterTimeConstant=0.001  UdotUserProvided=1
  Simulink-PS Converter12 : nesl_utility/Simulink-PS Converter  PhysicalDomain=network_engine_domain  SubClassName=ps_input  LeftPortType=input  RightPortType=output  PseudoPeriodic=off  Frequencies=[]  NoiseDistribution=none  NoiseParameters=[]  Unit=gal/min  AffineConversion=off  FilteringAndDerivatives=zero  SimscapeFilterOrder=1  InputFilterTimeConstant=0.001  UdotUserProvided=1
  Simulink-PS Converter4 : nesl_utility/Simulink-PS Converter  PhysicalDomain=network_engine_domain  SubClassName=ps_input  LeftPortType=input  RightPortType=output  PseudoPeriodic=off  Frequencies=[]  NoiseDistribution=none  NoiseParameters=[]  Unit=gal/min  AffineConversion=off  FilteringAndDerivatives=zero  SimscapeFilterOrder=1  InputFilterTimeConstant=0.001  UdotUserProvided=1
  Simulink-PS Converter8 : nesl_utility/Simulink-PS Converter  PhysicalDomain=network_engine_domain  SubClassName=ps_input  LeftPortType=input  RightPortType=output  PseudoPeriodic=off  Frequencies=[]  NoiseDistribution=none  NoiseParameters=[]  Unit=rpm  AffineConversion=off  FilteringAndDerivatives=zero  SimscapeFilterOrder=1  InputFilterTimeConstant=0.001  UdotUserProvided=1
  Unit Delay : UnitDelay  SampleTime=3
  Waste Flow : fl_lib/Hydraulic/Hydraulic Sources/Hydraulic Flow Rate Source
      settings: SourceProductName=Simscape  SourceProductBaseCode=SS
  p_hw_sensor : fl_lib/Hydraulic/Hydraulic Sensors/Hydraulic Pressure Sensor
      settings: SourceProductName=Simscape
  p_tank_sensor : fl_lib/Hydraulic/Hydraulic Sensors/Hydraulic Pressure Sensor
      settings: SourceProductName=Simscape
  recycle_tank_sensor : fl_lib/Hydraulic/Hydraulic Sensors/Hydraulic Pressure Sensor
      settings: SourceProductName=Simscape
  Rain Water Supply : PMIOPort  Port=1  Side=Left
  Potable Water Supply : PMIOPort  Port=2  Side=Right
  Recycle Water Supply : PMIOPort  Port=3  Side=Right
  Hot Water Supply : PMIOPort  Port=4  Side=Right
  tag scope: p_hw=global, p_tank=global, p_tank_recycle=global, vol_cistern=global, vol_grey_cistern=global
  wires:
  PS-Simulink Converter/1 -> [vol_cistern]  "vol_cistern"
  PS-Simulink Converter1/1 -> [p_tank]
  [filter_rain] -> Simulink-PS Converter2/1
  [cistern_valve] -> Simulink-PS Converter3/1
  [pump_speed] -> Simulink-PS Converter1/1
  [hw_valve] -> Simulink-PS Converter6/1
  [grey_pump_speed] -> Simulink-PS Converter8/1
  [filter_grey] -> Simulink-PS Converter9/1
  PS-Simulink Converter3/1 -> [p_tank_recycle]
  [grey_cistern_valve] -> Simulink-PS Converter10/1
  PS-Simulink Converter4/1 -> [vol_grey_cistern]  "vol_grey_cistern"
  Unit Delay/1 -> Simulink-PS Converter4/1
  [recycle_flowrate] -> Unit Delay/1
  [overflow_grey_valve] -> Simulink-PS Converter11/1
  PS-Simulink Converter5/1 -> Gain/1
  Gain/1 -> Simulink-PS Converter12/1  "waste_flow"
  [rain_flush_valve] -> Simulink-PS Converter5/1
  PS-Simulink Converter8/1 -> [p_hw]
  connections:
  Ideal Angular Velocity Source/LConn1 -- RainFlo MPH 75/LConn1
  Cistern/LConn1 -- Rain Water Supply/RConn1
  Simulink-PS Converter1/RConn1 -- Ideal Angular Velocity Source/RConn1
  Mechanical Rotational Reference/LConn1 -- Ideal Angular Velocity Source/RConn2
  Cistern/RConn1 -- PS-Simulink Converter/LConn1
  Hydraulic Reference/LConn1 -- p_tank_sensor/RConn1
  PS-Simulink Converter1/LConn1 -- p_tank_sensor/RConn2
  RainFlo MPH 75/RConn1 -- Pump Valve/LConn2
  Pump Valve/LConn1 -- Simulink-PS Converter2/RConn1
  Cistern Valve/LConn2 -- Cistern Valve1/LConn2 -- Cistern/RConn2
  RainFlo MPH 75/RConn2 -- Cistern Valve/RConn1
  Simulink-PS Converter3/RConn1 -- Cistern Valve/LConn1
  Pressure Tank Pipe/LConn1 -- Pump Valve/RConn1
  Rain Filter/LConn1 -- Pressure Tank Pipe/RConn1
  HW Valve/RConn1 -- Pressure Tank Pipe1/LConn1
  HW Valve/LConn1 -- Simulink-PS Converter6/RConn1
  Mechanical Rotational Reference1/LConn1 -- Ideal Angular Velocity Source1/RConn2
  Simulink-PS Converter8/RConn1 -- Ideal Angular Velocity Source1/RConn1
  Ideal Angular Velocity Source1/LConn1 -- Grey Water Pump/LConn1
  recycle_tank_sensor/LConn1 -- HW Valve/LConn2 -- Recycle Water Supply/RConn1 -- RO/RConn1 -- Recycle Pressure Tank/RConn1
  Grey Water Pump/RConn1 -- Grey Pump Valve/LConn2
  Simulink-PS Converter9/RConn1 -- Grey Pump Valve/LConn1
  PS-Simulink Converter3/LConn1 -- recycle_tank_sensor/RConn2
  Hydraulic Reference2/LConn1 -- recycle_tank_sensor/RConn1
  Grey Water Pump/RConn2 -- Grey Cistern Valve/RConn1
  Simulink-PS Converter10/RConn1 -- Grey Cistern Valve/LConn1
  Potable Pressure Tank/RConn1 -- p_tank_sensor/LConn1 -- Potable Water Supply/RConn1 -- Rain Filter/RConn1
  Grey Cistern/LConn1 -- Cistern Valve1/RConn1 -- Hydraulic Flow Rate Source/LConn1
  Grey Cistern/RConn1 -- PS-Simulink Converter4/LConn1
  Grey Cistern/RConn2 -- Grey Cistern Valve/LConn2 -- Overflow Valve/LConn2
  Hydraulic Reference3/LConn1 -- Hydraulic Flow Rate Source/RConn2
  Simulink-PS Converter4/RConn1 -- Hydraulic Flow Rate Source/RConn1
  RO Flow rate/RConn2 -- Waste Flow/RConn2 -- RO/LConn1
  Grey Pump Valve/RConn1 -- RO Flow rate/LConn1
  Overflow Valve/RConn1 -- Hydraulic Reference4/LConn1
  Simulink-PS Converter11/RConn1 -- Overflow Valve/LConn1
  PS-Simulink Converter5/LConn1 -- RO Flow rate/RConn1
  Simulink-PS Converter12/RConn1 -- Waste Flow/RConn1
  Hydraulic Reference5/LConn1 -- Waste Flow/LConn1
  Simulink-PS Converter5/RConn1 -- Cistern Valve1/LConn1
  Recycle Pressure Tank1/RConn1 -- Pressure Tank Pipe1/RConn1 -- p_hw_sensor/LConn1 -- RO Flow rate1/LConn1
  p_hw_sensor/RConn1 -- Hydraulic Reference1/LConn1
  PS-Simulink Converter8/LConn1 -- p_hw_sensor/RConn2
  Hot Water Supply/RConn1 -- RO Flow rate1/RConn2
  PS-Simulink Converter7/LConn1 -- RO Flow rate1/RConn1

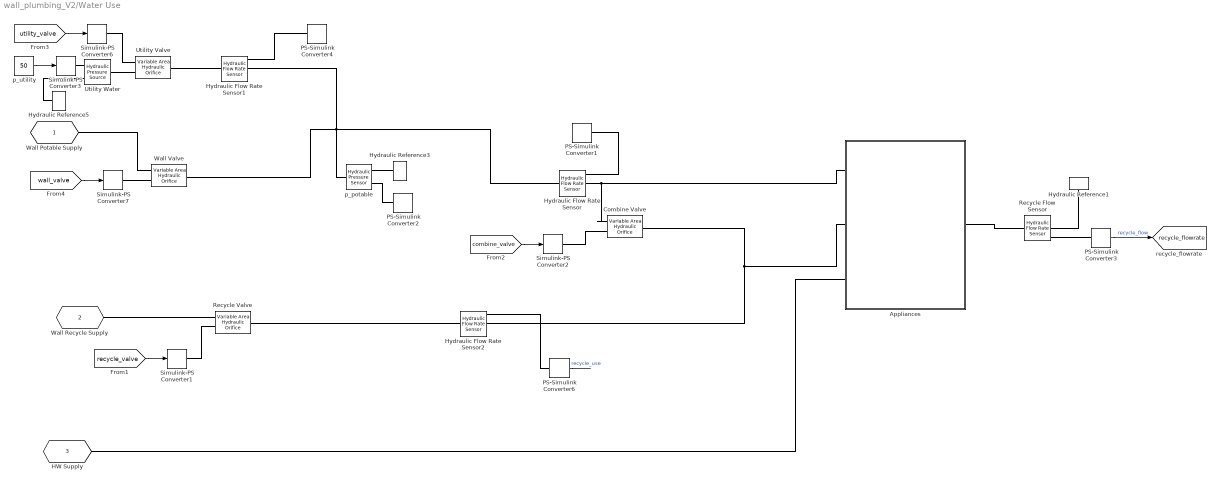
== system wall_plumbing_V2/Water Use ==
  Appliances : Subsystem
  Combine Valve : fl_lib/Hydraulic/Hydraulic Elements/Variable Area Hydraulic Orifice  C_d=0.7  min_area=1e-12 m^2  lam_spec=1  B_lam=0.999  Re_cr=12  q_specify=off  q_priority=None  q=0.001 m^3/s  q_nominal_specify=off  q_nominal_unit=m^3/s  q_nominal_value=1  p_specify=off  p_priority=None  p=0 Pa  p_nominal_specify=off  p_nominal_unit=Pa  p_nominal_value=1
      settings: SourceProductName=Simscape  SourceProductBaseCode=SS
  Hydraulic Flow Rate Sensor : fl_lib/Hydraulic/Hydraulic Sensors/Hydraulic Flow Rate Sensor
      settings: SourceProductName=Simscape
  Hydraulic Flow Rate Sensor1 : fl_lib/Hydraulic/Hydraulic Sensors/Hydraulic Flow Rate Sensor
      settings: SourceProductName=Simscape
  Hydraulic Flow Rate Sensor2 : fl_lib/Hydraulic/Hydraulic Sensors/Hydraulic Flow Rate Sensor
      settings: SourceProductName=Simscape
  Hydraulic Reference1 : fl_lib/Hydraulic/Hydraulic Elements/Hydraulic Reference
      settings: SourceProductName=Simscape
  Hydraulic Reference3 : fl_lib/Hydraulic/Hydraulic Elements/Hydraulic Reference
      settings: SourceProductName=Foundation Library
  Hydraulic Reference5 : fl_lib/Hydraulic/Hydraulic Elements/Hydraulic Reference
      settings: SourceProductName=Foundation Library
  PS-Simulink Converter{1,3..4,6} (4 alike) : nesl_utility/PS-Simulink Converter  PhysicalDomain=network_engine_domain  SubClassName=ps_output  LeftPortType=input  RightPortType=output  PseudoPeriodic=off  Frequencies=[]  Unit=gal/min  AffineConversion=off
  PS-Simulink Converter2 : nesl_utility/PS-Simulink Converter  PhysicalDomain=network_engine_domain  SubClassName=ps_output  LeftPortType=input  RightPortType=output  PseudoPeriodic=off  Frequencies=[]  Unit=psi  AffineConversion=off
  Recycle Flow Sensor : fl_lib/Hydraulic/Hydraulic Sensors/Hydraulic Flow Rate Sensor
      settings: SourceProductName=Simscape
  Recycle Valve : fl_lib/Hydraulic/Hydraulic Elements/Variable Area Hydraulic Orifice  C_d=0.7  min_area=1e-12 m^2  lam_spec=1  B_lam=0.999  Re_cr=12  q_specify=off  q_priority=None  q=0.001 m^3/s  q_nominal_specify=off  q_nominal_unit=m^3/s  q_nominal_value=1  p_specify=off  p_priority=None  p=0 Pa  p_nominal_specify=off  p_nominal_unit=Pa  p_nominal_value=1
      settings: SourceProductName=Simscape  SourceProductBaseCode=SS
  Simulink-PS Converter{1..2,6..7} (4 alike) : nesl_utility/Simulink-PS Converter  PhysicalDomain=network_engine_domain  SubClassName=ps_input  LeftPortType=input  RightPortType=output  PseudoPeriodic=off  Frequencies=[]  NoiseDistribution=none  NoiseParameters=[]  Unit=in^2  AffineConversion=off  FilteringAndDerivatives=zero  SimscapeFilterOrder=1  InputFilterTimeConstant=0.001  UdotUserProvided=1
  Simulink-PS Converter3 : nesl_utility/Simulink-PS Converter  PhysicalDomain=network_engine_domain  SubClassName=ps_input  LeftPortType=input  RightPortType=output  PseudoPeriodic=off  Frequencies=[]  NoiseDistribution=none  NoiseParameters=[]  Unit=1  AffineConversion=off  FilteringAndDerivatives=zero  SimscapeFilterOrder=1  InputFilterTimeConstant=0.001  UdotUserProvided=1
  Utility Valve : fl_lib/Hydraulic/Hydraulic Elements/Variable Area Hydraulic Orifice  C_d=0.7  min_area=1e-12 m^2  lam_spec=1  B_lam=0.999  Re_cr=12  q_specify=off  q_priority=None  q=0.001 m^3/s  q_nominal_specify=off  q_nominal_unit=m^3/s  q_nominal_value=1  p_specify=off  p_priority=None  p=0 Pa  p_nominal_specify=off  p_nominal_unit=Pa  p_nominal_value=1
      settings: SourceProductName=Simscape  SourceProductBaseCode=SS
  Utility Water : fl_lib/Hydraulic/Hydraulic Sources/Hydraulic Pressure Source
      settings: SourceProductName=Simscape  SourceProductBaseCode=SS
  Wall Valve : fl_lib/Hydraulic/Hydraulic Elements/Variable Area Hydraulic Orifice  C_d=0.7  min_area=1e-12 m^2  lam_spec=1  B_lam=0.999  Re_cr=12  q_specify=off  q_priority=None  q=0.001 m^3/s  q_nominal_specify=off  q_nominal_unit=m^3/s  q_nominal_value=1  p_specify=off  p_priority=None  p=0 Pa  p_nominal_specify=off  p_nominal_unit=Pa  p_nominal_value=1
      settings: SourceProductName=Simscape  SourceProductBaseCode=SS
  p_potable : fl_lib/Hydraulic/Hydraulic Sensors/Hydraulic Pressure Sensor
      settings: SourceProductName=Simscape
  p_utility : Constant  Value=50
  Wall Potable Supply : PMIOPort  Port=1  Side=Left
  Wall Recycle Supply : PMIOPort  Port=2  Side=Left
  HW Supply : PMIOPort  Port=3  Side=Left
  tag scope: recycle_flowrate=global
  wires:
  p_utility/1 -> Simulink-PS Converter3/1
  [utility_valve] -> Simulink-PS Converter6/1
  [wall_valve] -> Simulink-PS Converter7/1
  [recycle_valve] -> Simulink-PS Converter1/1
  [combine_valve] -> Simulink-PS Converter2/1
  PS-Simulink Converter3/1 -> [recycle_flowrate]  "recycle_flow"
  PS-Simulink Converter6/1 -> ?  "recycle_use"
  connections:
  Utility Water/RConn2 -- Hydraulic Reference5/LConn1
  Simulink-PS Converter3/RConn1 -- Utility Water/RConn1
  p_potable/RConn2 -- PS-Simulink Converter2/LConn1
  Simulink-PS Converter6/RConn1 -- Utility Valve/LConn1
  Utility Valve/LConn2 -- Utility Water/LConn1
  Simulink-PS Converter7/RConn1 -- Wall Valve/LConn1
  Wall Valve/RConn1 -- Hydraulic Flow Rate Sensor1/RConn2 -- Hydraulic Flow Rate Sensor/LConn1 -- p_potable/LConn1
  Hydraulic Flow Rate Sensor/RConn1 -- PS-Simulink Converter1/LConn1
  PS-Simulink Converter3/LConn1 -- Recycle Flow Sensor/RConn1
  Wall Potable Supply/RConn1 -- Wall Valve/LConn2
  Hydraulic Reference3/LConn1 -- p_potable/RConn1
  Hydraulic Flow Rate Sensor/RConn2 -- Appliances/LConn1 -- Combine Valve/LConn2
  Appliances/RConn1 -- Recycle Flow Sensor/LConn1
  Hydraulic Reference1/LConn1 -- Recycle Flow Sensor/RConn2
  Simulink-PS Converter1/RConn1 -- Recycle Valve/LConn1
  Recycle Valve/LConn2 -- Wall Recycle Supply/RConn1
  Combine Valve/RConn1 -- Appliances/LConn2 -- Hydraulic Flow Rate Sensor2/RConn2
  Simulink-PS Converter2/RConn1 -- Combine Valve/LConn1
  Hydraulic Flow Rate Sensor2/LConn1 -- Recycle Valve/RConn1
  PS-Simulink Converter6/LConn1 -- Hydraulic Flow Rate Sensor2/RConn1
  Utility Valve/RConn1 -- Hydraulic Flow Rate Sensor1/LConn1
  Hydraulic Flow Rate Sensor1/RConn1 -- PS-Simulink Converter4/LConn1
  Appliances/LConn3 -- HW Supply/RConn1
